simulink model "SF019B_PwrLimr"  (R2013b)
settings: Solver=FixedStepDiscrete  SolverMode=SingleTasking  StartTime=0.0  StopTime=1  FixedStep=0.002  RelTol=1e-3
values from neighbouring files (symbols this model uses):
  ARCHGLBPRM_2MILLISEC_SEC_F32 = DataDict.Constant    [SF019B_PwrLimr_DataDict.m]
  ELECGLBPRM_IVTRCNT_CNT_U08 = DataDict.ConfigParam    [SF019B_PwrLimr_DataDict.m]
  PwrLimrBackEmfConStdT = DataDict.Calibration    [SF019B_PwrLimr_DataDict.m]
  PwrLimrBrdgVltgAdjSlew = DataDict.Calibration    [SF019B_PwrLimr_DataDict.m]
  PwrLimrBrdgVltgAltFltAdj = DataDict.Calibration    [SF019B_PwrLimr_DataDict.m]
  PwrLimrFilAssiRednThd = DataDict.Calibration    [SF019B_PwrLimr_DataDict.m]
  PwrLimrLoVoltAssiRcvrThd = DataDict.Calibration    [SF019B_PwrLimr_DataDict.m]
  PwrLimrLoVoltAssiRcvrTi = DataDict.Calibration    [SF019B_PwrLimr_DataDict.m]
  PWRLIMRMILLISECTOSEC_SECPERMILLISEC_F32 = DataDict.Constant    [SF019B_PwrLimr_DataDict.m]
  PwrLimrMotEnvlpX = DataDict.Calibration    [SF019B_PwrLimr_DataDict.m]
  PwrLimrMotEnvlpY = DataDict.Calibration    [SF019B_PwrLimr_DataDict.m]
  PwrLimrSpdAdjSlewDec = DataDict.Calibration    [SF019B_PwrLimr_DataDict.m]
  PwrLimrSpdAdjSlewEna = DataDict.Calibration    [SF019B_PwrLimr_DataDict.m]
  PwrLimrSpdAdjSlewInc = DataDict.Calibration    [SF019B_PwrLimr_DataDict.m]
  PwrLimrStdOperMotEnvlpX = DataDict.Calibration    [SF019B_PwrLimr_DataDict.m]
  PwrLimrStdOperMotEnvlpY = DataDict.Calibration    [SF019B_PwrLimr_DataDict.m]
  PwrLimrVltgDptMotVelOffsX = DataDict.Calibration    [SF019B_PwrLimr_DataDict.m]
  PwrLimrVltgDptMotVelOffsY = DataDict.Calibration    [SF019B_PwrLimr_DataDict.m]
undefined symbols (not defined in the file or in its folder): D_2MS_SEC_F32
undefined symbols (not defined in the file): ARCHGLBPRM_10MILLISEC_SEC_F32, PwrLimrAssiRednLpFilFrq, PwrLimrMotVelLpFilFrq
libraries: simulink x12, NxtrLim x2
(part 1 of 2)
settings Model: Creator=szj6ld  LastModifiedBy=RZ2YLP
settings SolverCC: AutoInsertRateTranBlk=on  InsertRTBMode=Always
settings DataIOCC: LimitDataPoints=off  SaveFormat=Structure  ReturnWorkspaceOutputs=on
settings OptimizationCC: BlockReduction=off  InlineParams=on  ZeroExternalMemoryAtStartup=off  ZeroInternalMemoryAtStartup=off  OptimizeModelRefInitCode=on  LifeSpan=1
settings DebuggingCC: SignalInfNanChecking=error  SignalRangeChecking=warning  UnderspecifiedInitializationDetection=Simplified  SolverPrmCheckMsg=error  InheritedTsInSrcMsg=error  DiscreteInheritContinuousMsg=error  SingleTaskRateTransMsg=error  TasksWithSamePriorityMsg=error  SigSpecEnsureSampleTimeMsg=error  CheckMatrixSingularityMsg=error  ParameterUnderflowMsg=error  ParameterPrecisionLossMsg=error  ParameterTunabilityLossMsg=error  FixptConstUnderflowMsg=warning  FixptConstOverflowMsg=warning  VectorMatrixConversionMsg=error  SignalLabelMismatchMsg=error  UnconnectedInputMsg=error  UnconnectedOutputMsg=error  UnconnectedLineMsg=error  SFcnCompatibilityMsg=error  UniqueDataStoreMsg=warning  BusObjectLabelMismatch=error  RootOutportRequireBusObject=error  AssertControl=DisableAll  ModelReferenceIOMsg=error  ModelReferenceVersionMismatchMessage=warning  ModelReferenceIOMismatchMessage=error  ModelReferenceCSMismatchMessage=warning  ModelReferenceDataLoggingMessage=error  StateNameClashWarn=warning  StrictBusMsg=ErrorOnBusTreatedAsVector  NonBusSignalsTreatedAsBus=error  SFUnexpectedBacktrackingDiag=error  SFInvalidInputDataAccessInChartInitDiag=error  SFNoUnconditionalDefaultTransitionDiag=error  SFTransitionOutsideNaturalParentDiag=error  SFUnconditionalTransitionShadowingDiag=error  SFUndirectedBroadcastEventsDiag=error
settings ModelReferenceCC: ModelReferenceNumInstancesAllowed=Single
settings RTWCC: SystemTargetFile=autosar.tlc  GenCodeOnly=on  TemplateMakefile=ert_default_tmf  Description=AUTOSAR  GenerateReport=on  ProcessScript=autosar_make_rtw_hook  LaunchReport=on
settings CodeAppCC: GenerateComments=off  IgnoreCustomStorageClasses=off  CustomSymbolStrType=$N$R$M  CustomSymbolStrBlkIO=$N$M  SimulinkBlockComments=off
settings STFCustomTargetCC: ParMdlRefBuildCompliant=on  CompOptLevelCompliant=on  IncludeMdlTerminateFcn=off  CombineOutputUpdateFcns=on  SuppressErrorStatus=on  ERTFirstTimeCompliant=on  ERTCustomFileBanners=on  SupportNonFinite=off  SupportComplex=off  SupportContinuousTime=off  SupportNonInlinedSFcns=off  MATLABClassNameForMDSCustomization=Simulink.SoftwareTarget.ERTCustomization  AutosarCompliant=on  GRTInterface=off  SystemTargetFile=autosar.tlc
settings ERTTargetCC: CodeReplacementLibrary=ANSI_C  ConcurrentExecutionCompliant=off  IncludeMdlTerminateFcn=off  SuppressErrorStatus=on  SupportNonFinite=off  SupportComplex=off  ModelStepFunctionPrototypeControlCompliant=off  CPPClassGenCompliant=off  AutosarCompliant=on  InlinedParameterPlacement=NonHierarchical  ERTCustomFileTemplate=example_file_process.tlc  EnableUserReplacementTypes=on

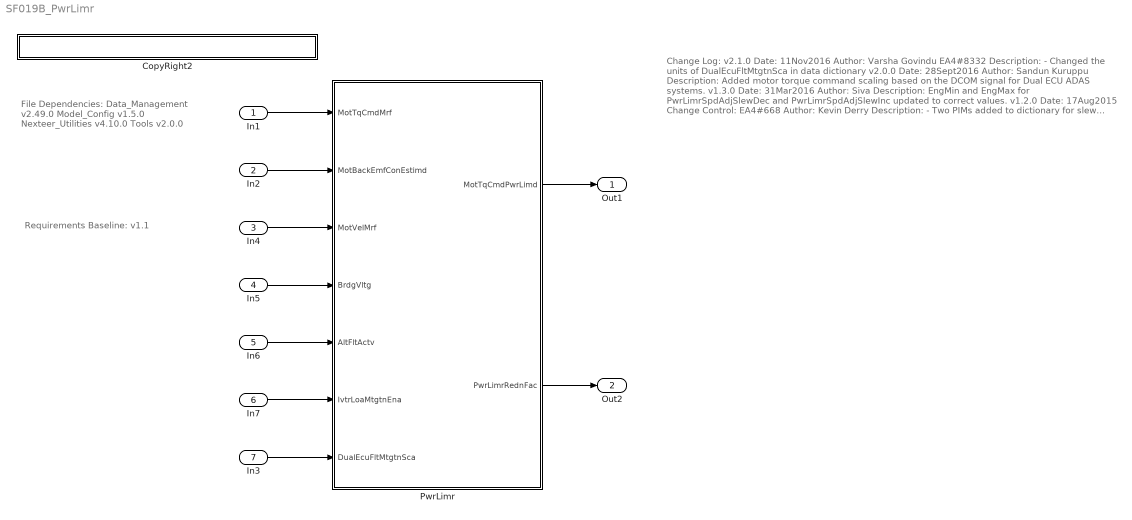
== system SF019B_PwrLimr ==
  note: Requirements Baseline: v1.1
  note: File Dependencies:
      |
      | Data_Management v2.49.0
      | Model_Config v1.5.0
      | Nexteer_Utilities v4.10.0
      | Tools v2.0.0
  note: Change Log:
      |
      | v2.1.0
      | Date: 11Nov2016
      | Author: Varsha Govindu
      | EA4#8332
      | Description:
      | - Changed the units of DualEcuFltMtgtnSca in data dictionary
      |
      | v2.0.0
      | Date: 28Sept2016
      | Author: Sandun Kuruppu
      | Description:
      | Added motor torque command scaling based on the DCOM signal for Dual ECU ADAS systems.
      |
      | v1.3.0
      | Date: 31Mar2016
      | Author: Siva
      | Description:
      | EngMin and EngMax for PwrLimrSpdAdjSlewDec and PwrLimrSpdAdjSlewInc updated to correct values.
      |
      | v1.2.0
      | Date:  17Aug2015
      | Change Control:  EA4#668
      | Author:  Kevin Derry
      | Description:
      | -  Two PIMs added to dictionary for slew operations
      | -  Saturation block added to Per1 output.
      | -  Saturation block added to Per2 output.
      | -  PWRLIMRTQLIMHILIM_CNT_LGC  is now ULS_F32
      | -  PWRLIMRTQLIMLOLIM_CNT_LGC  is now ULS_F32
      | -  Cal PwrLimrVltgDptMotVelOffsY.EngMax was 1350, now 695 to match EA3.
      |
      | v1.1.0
      | Date:  14Aug2015
      | Change Control: EA4#668
      | Author:  Kevin Derry
      | Description:
      | -  Three IRVs added to dictionary
      | -  One PIM added to dictionary for fault timer.
      | -  Timer-related clients added to dictionary.
      | -  Corrected Change Control number in v1.0.0 below.
      |
      |
      | V1.0.0
      | Date: 04AUG2015
      | Change Control: EA4#668
      | Author: Chris Wheatley
      | Description:
      | - Initial Release in EA4
      | - Based on Revision 11.0.0 in EA3
      | - This is a level 0 design model and as such
      |   used only for reference.
  In1 : Inport
  In2 : Inport  Port=2
  In4 : Inport  Port=3
  In5 : Inport  Port=4
  In6 : Inport  Port=5
  In7 : Inport  Port=6
  In3 : Inport  Port=7
  CopyRight2 : Subsystem  Description=|  mask(Copyright Information){none=on}
      | Copyright info block.                                               
      |                                                                     
      | Place copyright information at the top of every subsystem in design.
      mask prompts: none "No parameters"
      mask help: Place copyright information at the top of every subsystem in design.
      mask Display:
      | NxtrConf = 'Nexteer Confidential';
      | 
      | sys = bdroot; %handle for the current model ("system")
      | first = get_param(sys,'Created');
      | first = first(end-3:end);  %year is last four digits
      | 
      | last = get_param(sys,'LastModifiedDate');
      | if isempty(last)
      |     last = datestr(now,'yyyy');
      | else
      |     last = last(end-3:end);
      | end
      | 
      | if strcmp(first,last)
      |     fprintf('%s -- Copyright %s Nexteer',NxtrConf,first)
      | else
      |     fprintf('%s -- %s%s- %s Nexteer',NxtrConf,char(169),first,last)
      | end
  PwrLimr : Subsystem  RequirementInfo="{'linktype_rmi_doors' '0000a532 (/E-STEER Core/SubSystem Specifications/Application Functions/SF019B Power Limit Function- Current Mode)' '#SF019B_245' 'true' 'REQ:  SF019B_245' '' ; 'linktype_rmi_doors' '0000a532 (/E-STEER Core/SubSystem Specifications/Application Functions/SF019B Power Limit Function- Current Mode)' '#SF019B_9' 'true' 'REQ:  SF019B_9' '' ; 'linktype_rmi_doors' '0000a532 (/E-STEER Core/SubSystem Specifications/Application Functions/SF019B Power Limit Function- Current Mode)' '#SF019B_32' 'true' 'REQ:  SF019B_32' '' ; 'linktype_rmi_doors' '0000a532 (/E-STEER Core/SubSystem Specifications/Application Functions/SF019B Power Limit Function- Current Mode)' '#SF019B_33' 'true' 'REQ:  SF019B_33' '' ; 'linktype_rmi_doors' '0000a532 (/E-STEER Core/SubSystem Specifications/Application Functions/SF019B Power Limit Function- Current Mode)' '#SF019B_34' 'true' 'REQ:  SF019B_34' '' ; 'linktype_rmi_doors' '0000a532 (/E-STEER Core/SubSystem Specifications/Application Functions/SF019B Power Limit Function- Current Mode)' '#SF019B_35' 'true' 'REQ:  SF019B_35' '' ; 'linktype_rmi_doors' '0000a532 (/E-STEER Core/SubSystem Specifications/Application Functions/SF019B Power Limit Function- Current Mode)' '#SF019B_36' 'true' 'REQ:  SF019B_36' '' ; 'linktype_rmi_doors' '0000a532 (/E-STEER Core/SubSystem Specifications/Application Functions/SF019B Power Limit Function- Current Mode)' '#SF019B_250' 'true' 'REQ:  SF019B_250' '' ; 'linktype_rmi_doors' '0000a532 (/E-STEER Core/SubSystem Specifications/Application Functions/SF019B Power Limit Function- Current Mode)' '#SF019B_11' 'true' 'REQ:  SF019B_11' '' ; 'linktype_rmi_doors' '0000a532 (/E-STEER Core/SubSystem Specifications/Application Functions/SF019B Power Limit Function- Current Mode)' '#SF019B_37' 'true' 'REQ:  SF019B_37' '' } %GIDa_deb22b8e_5f7e_4de5_8336_875e20a00c31"
  Out1 : Outport
  Out2 : Outport  Port=2
  wires:
  In1/1 -> PwrLimr/1(MotTqCmdMrf)
  In2/1 -> PwrLimr/2(MotBackEmfConEstimd)
  In4/1 -> PwrLimr/3(MotVelMrf)
  In5/1 -> PwrLimr/4(BrdgVltg)
  In6/1 -> PwrLimr/5(AltFltActv)
  In7/1 -> PwrLimr/6(IvtrLoaMtgtnEna)
  PwrLimr/1(MotTqCmdPwrLimd) -> Out1/1
  PwrLimr/2(PwrLimrRednFac) -> Out2/1
  In3/1 -> PwrLimr/7(DualEcuFltMtgtnSca)

== system SF019B_PwrLimr/CopyRight2 ==

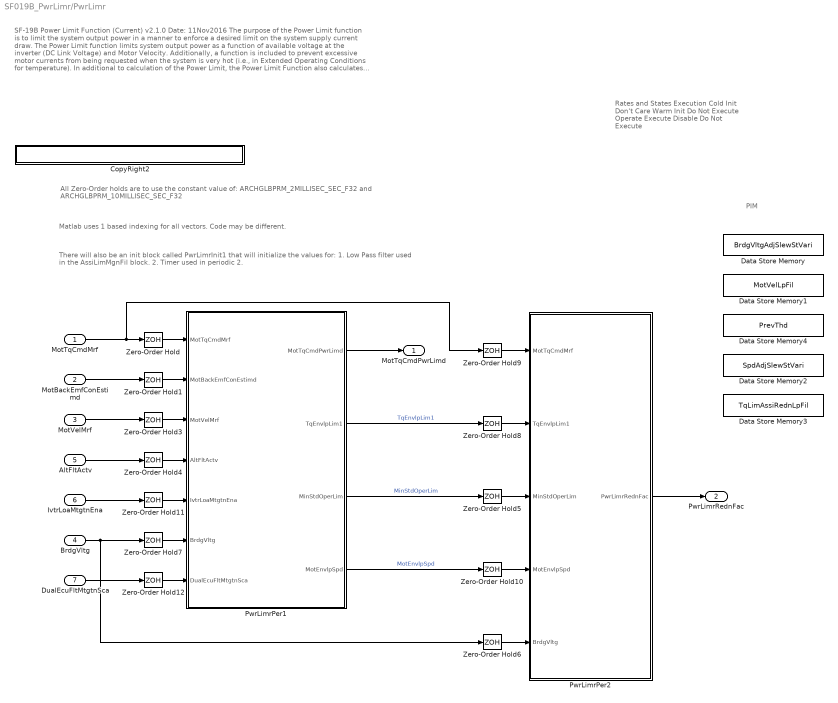
== system SF019B_PwrLimr/PwrLimr ==
  note: Matlab uses 1 based indexing for all vectors. Code may be different.
  note: There will also be an init block called PwrLimrInit1 that will initialize the values for:
      |    1. Low Pass filter used in the AssiLimMgnFil block.
      |    2. Timer used in periodic 2.
  note: SF-19B Power Limit Function (Current)
      | v2.1.0 Date: 11Nov2016
      |
      | The purpose of the Power Limit function is to limit the system output  power in a manner to enforce a desired limit on the system supply current draw.
      | The Power Limit function limits system output power as a function of available voltage at the inverter (DC Link Voltage) and Motor Velocity.  Additionally,
      | a function is included to prevent excessive  motor currents from being requested when the system is very hot (i.e., in Extended Operating Conditions
      | for temperature).
      | In additional to calculation of the Power Limit, the Power Limit Function  also calculates a level of degradation from Standard Operating Conditions full
      | performance and sets flags appropriately for a DTC (Log Only).
  note: Rates and States Execution
      |   Cold Init     Don't Care
      |   Warm Init   Do Not Execute
      |   Operate     Execute
      |   Disable      Do Not Execute
  note: All Zero-Order holds are to use the constant value of:
      | ARCHGLBPRM_2MILLISEC_SEC_F32 and  ARCHGLBPRM_10MILLISEC_SEC_F32
  note: PIM
  MotTqCmdMrf : Inport  RequirementInfo="{}  %GIDa_a11c376a_47bf_4292_9658_09aa228911af"
  MotBackEmfConEstimd : Inport  Port=2
  MotVelMrf : Inport  Port=3
  BrdgVltg : Inport  Port=4
  AltFltActv : Inport  Port=5
  IvtrLoaMtgtnEna : Inport  Port=6
  DualEcuFltMtgtnSca : Inport  Port=7
  CopyRight2 : Subsystem  Description=|  mask(Copyright Information){none=on}
      | Copyright info block.                                               
      |                                                                     
      | Place copyright information at the top of every subsystem in design.
      mask prompts: none "No parameters"
      mask help: Place copyright information at the top of every subsystem in design.
      mask Display:
      | NxtrConf = 'Nexteer Confidential';
      | 
      | sys = bdroot; %handle for the current model ("system")
      | first = get_param(sys,'Created');
      | first = first(end-3:end);  %year is last four digits
      | 
      | last = get_param(sys,'LastModifiedDate');
      | if isempty(last)
      |     last = datestr(now,'yyyy');
      | else
      |     last = last(end-3:end);
      | end
      | 
      | if strcmp(first,last)
      |     fprintf('%s -- Copyright %s Nexteer',NxtrConf,first)
      | else
      |     fprintf('%s -- %s%s- %s Nexteer',NxtrConf,char(169),first,last)
      | end
  Data Store Memory : DataStoreMemory  DataStoreName=BrdgVltgAdjSlewStVari  ReadBeforeWriteMsg=warning  WriteAfterWriteMsg=warning  WriteAfterReadMsg=warning  StateMustResolveToSignalObject=on
  Data Store Memory1 : DataStoreMemory  DataStoreName=MotVelLpFil  ReadBeforeWriteMsg=warning  WriteAfterWriteMsg=warning  WriteAfterReadMsg=warning  InitialValue=[]  OutDataTypeStr=Bus: FilLpRec1  StateMustResolveToSignalObject=on
  Data Store Memory2 : DataStoreMemory  DataStoreName=SpdAdjSlewStVari  ReadBeforeWriteMsg=warning  WriteAfterWriteMsg=warning  WriteAfterReadMsg=warning  StateMustResolveToSignalObject=on
  Data Store Memory3 : DataStoreMemory  DataStoreName=TqLimAssiRednLpFil  ReadBeforeWriteMsg=warning  WriteAfterWriteMsg=warning  WriteAfterReadMsg=warning  InitialValue=[]  OutDataTypeStr=Bus: FilLpRec1  StateMustResolveToSignalObject=on
  Data Store Memory4 : DataStoreMemory  DataStoreName=PrevThd  ReadBeforeWriteMsg=warning  WriteAfterWriteMsg=warning  WriteAfterReadMsg=warning  StateMustResolveToSignalObject=on
  PwrLimrPer1 : Subsystem  RequirementInfo="{'linktype_rmi_doors' '0000a532 (/E-STEER Core/SubSystem Specifications/Application Functions/SF019B Power Limit Function- Current Mode)' '#SF019B_197' 'true' 'REQ:  SF019B_197' '' ; 'linktype_rmi_doors' '0000a532 (/E-STEER Core/SubSystem Specifications/Application Functions/SF019B Power Limit Function- Current Mode)' '#SF019B_198' 'true' 'REQ:  SF019B_198' '' ; 'linktype_rmi_doors' '0000a532 (/E-STEER Core/SubSystem Specifications/Application Functions/SF019B Power Limit Function- Current Mode)' '#SF019B_199' 'true' 'REQ:  SF019B_199' '' ; 'linktype_rmi_doors' '0000a532 (/E-STEER Core/SubSystem Specifications/Application Functions/SF019B Power Limit Function- Current Mode)' '#SF019B_200' 'true' 'REQ:  SF019B_200' '' ; 'linktype_rmi_doors' '0000a532 (/E-STEER Core/SubSystem Specifications/Application Functions/SF019B Power Limit Function- Current Mode)' '#SF019B_254' 'true' 'REQ:  SF019B_254' '' ; 'linktype_rmi_doors' '0000a532 (/E-STEER Core/SubSystem Specifications/Application Functions/SF019B Power Limit Function- Current Mode)' '#SF019B_192' 'true' 'REQ:  SF019B_192' '' } %GIDa_bc7142bf_0b54_4f48_97b6_48859e905753"
  PwrLimrPer2 : Subsystem  RequirementInfo="{'linktype_rmi_doors' '0000a532 (/E-STEER Core/SubSystem Specifications/Application Functions/SF019B Power Limit Function- Current Mode)' '#SF019B_193' 'true' 'REQ:  SF019B_193' '' } %GIDa_9316d20a_733a_4c44_a986_53eaf77b60cd"
  Zero-Order Hold{,1,3..11} (11 alike) : ZeroOrderHold  SampleTime=-1
  Zero-Order Hold12 : ZeroOrderHold  SampleTime=D_2MS_SEC_F32
  MotTqCmdPwrLimd : Outport
  PwrLimrRednFac : Outport  Port=2
  wires:
  PwrLimrPer1/1(MotTqCmdPwrLimd) -> MotTqCmdPwrLimd/1
  PwrLimrPer1/3(MinStdOperLim) -> Zero-Order Hold5/1  "MinStdOperLim"
  MotBackEmfConEstimd/1 -> Zero-Order Hold1/1
  PwrLimrPer2/1(PwrLimrRednFac) -> PwrLimrRednFac/1
  MotVelMrf/1 -> Zero-Order Hold3/1
  BrdgVltg/1 -> Zero-Order Hold7/1, Zero-Order Hold6/1
  Zero-Order Hold1/1 -> PwrLimrPer1/2(MotBackEmfConEstimd)
  Zero-Order Hold3/1 -> PwrLimrPer1/3(MotVelMrf)
  Zero-Order Hold7/1 -> PwrLimrPer1/6(BrdgVltg)
  Zero-Order Hold9/1 -> PwrLimrPer2/1(MotTqCmdMrf)
  Zero-Order Hold8/1 -> PwrLimrPer2/2(TqEnvlpLim1)
  Zero-Order Hold5/1 -> PwrLimrPer2/3(MinStdOperLim)
  Zero-Order Hold6/1 -> PwrLimrPer2/5(BrdgVltg)
  Zero-Order Hold/1 -> PwrLimrPer1/1(MotTqCmdMrf)
  MotTqCmdMrf/1 -> Zero-Order Hold9/1, Zero-Order Hold/1
  Zero-Order Hold10/1 -> PwrLimrPer2/4(MotEnvlpSpd)
  PwrLimrPer1/4(MotEnvlpSpd) -> Zero-Order Hold10/1  "MotEnvlpSpd"
  PwrLimrPer1/2(TqEnvlpLim1) -> Zero-Order Hold8/1  "TqEnvlpLim1"
  AltFltActv/1 -> Zero-Order Hold4/1
  Zero-Order Hold4/1 -> PwrLimrPer1/4(AltFltActv)
  IvtrLoaMtgtnEna/1 -> Zero-Order Hold11/1
  Zero-Order Hold11/1 -> PwrLimrPer1/5(IvtrLoaMtgtnEna)
  Zero-Order Hold12/1 -> PwrLimrPer1/7(DualEcuFltMtgtnSca)
  DualEcuFltMtgtnSca/1 -> Zero-Order Hold12/1

== system SF019B_PwrLimr/PwrLimr/CopyRight2 ==

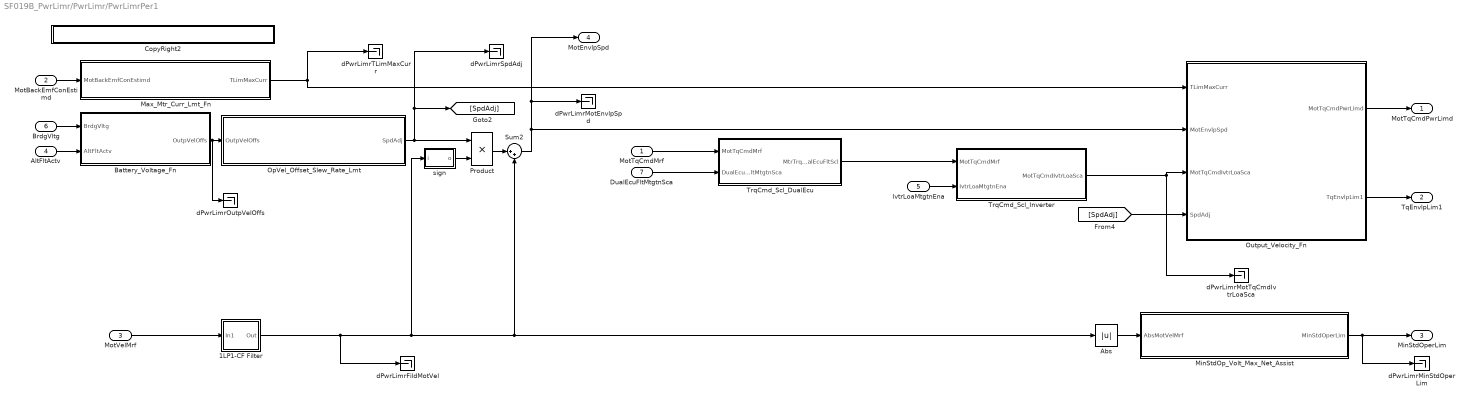
== system SF019B_PwrLimr/PwrLimr/PwrLimrPer1 ==
  MotTqCmdMrf : Inport
  MotBackEmfConEstimd : Inport  Port=2
  MotVelMrf : Inport  Port=3
  AltFltActv : Inport  Port=4
  IvtrLoaMtgtnEna : Inport  Port=5
  BrdgVltg : Inport  Port=6
  DualEcuFltMtgtnSca : Inport  Port=7
  1LP1-CF Filter : Subsystem  RequirementInfo="{'linktype_rmi_doors' '0000a532 (/E-STEER Core/SubSystem Specifications/Application Functions/SF019B Power Limit Function- Current Mode)' '#SF019B_130' 'true' 'REQ:  SF019B_130' '' ; 'linktype_rmi_doors' '0000a532 (/E-STEER Core/SubSystem Specifications/Application Functions/SF019B Power Limit Function- Current Mode)' '#SF019B_131' 'true' 'REQ:  SF019B_131' '' } %GIDa_0c73a69f_0b65_451d_a3dd_7bbd8b392771"  mask(1LP1-CF Filter){Ts=ARCHGLBPRM_2MILLISEC_SEC_F32, Kn_Hz=PwrLimrMotVelLpFilFrq, IC=0}
      mask prompts: Ts "Function Time Step (seconds)"; Kn_Hz "Cutoff Frequency in Hz"; IC "Initial Condition (Enineering Units)"
      mask help: version: Jun 14, 2012
      mask init:
      | %Convert cutoff frequency from Hz into floating point "counts"
      | Kn_Cnt = 1-exp(-2*pi*Kn_Hz*Ts);
      | 
      | %Filter design document originally called this value Knum
      | Knum = Kn_Cnt;
      settings: AttributesFormatString=%<Kn_Hz>
      mask Display:
      | port_label('input',1,'y')
      | disp 'LPF'
      | 
      | %a = [2:0.1:5.2]';
      | %b = sin(2*a);
      | %c = 0.7*sin(25*a);
      | %d = b+c;
      | %e = vertcat(d, b);
      | %plot(e);
  Abs : Abs
  Battery_Voltage_Fn : Subsystem  RequirementInfo="{'linktype_rmi_doors' '0000a532 (/E-STEER Core/SubSystem Specifications/Application Functions/SF019B Power Limit Function- Current Mode)' '#SF019B_64' 'true' 'REQ:  SF019B_64' '' ; 'linktype_rmi_doors' '0000a532 (/E-STEER Core/SubSystem Specifications/Application Functions/SF019B Power Limit Function- Current Mode)' '#SF019B_71' 'true' 'REQ:  SF019B_71' '' ; 'linktype_rmi_doors' '0000a532 (/E-STEER Core/SubSystem Specifications/Application Functions/SF019B Power Limit Function- Current Mode)' '#SF019B_202' 'true' 'REQ:  SF019B_202' '' } %GIDa_d1728748_224a_4c27_968a_5f2e6b163336"
  CopyRight2 : Subsystem  Description=|  mask(Copyright Information){none=on}
      | Copyright info block.                                               
      |                                                                     
      | Place copyright information at the top of every subsystem in design.
      mask prompts: none "No parameters"
      mask help: Place copyright information at the top of every subsystem in design.
      mask Display:
      | NxtrConf = 'Nexteer Confidential';
      | 
      | sys = bdroot; %handle for the current model ("system")
      | first = get_param(sys,'Created');
      | first = first(end-3:end);  %year is last four digits
      | 
      | last = get_param(sys,'LastModifiedDate');
      | if isempty(last)
      |     last = datestr(now,'yyyy');
      | else
      |     last = last(end-3:end);
      | end
      | 
      | if strcmp(first,last)
      |     fprintf('%s -- Copyright %s Nexteer',NxtrConf,first)
      | else
      |     fprintf('%s -- %s%s- %s Nexteer',NxtrConf,char(169),first,last)
      | end
  Max_Mtr_Curr_Lmt_Fn : Subsystem  RequirementInfo="{'linktype_rmi_doors' '0000a532 (/E-STEER Core/SubSystem Specifications/Application Functions/SF019B Power Limit Function- Current Mode)' '#SF019B_223' 'true' 'REQ:  SF019B_223' '' ; 'linktype_rmi_doors' '0000a532 (/E-STEER Core/SubSystem Specifications/Application Functions/SF019B Power Limit Function- Current Mode)' '#SF019B_228' 'true' 'REQ:  SF019B_228' '' } %GIDa_6b055ca6_9043_4c99_8b1e_e40a2fd42a97"
  MinStdOp_Volt_Max_Net_Assist : Subsystem  RequirementInfo="{'linktype_rmi_doors' '0000a532 (/E-STEER Core/SubSystem Specifications/Application Functions/SF019B Power Limit Function- Current Mode)' '#SF019B_181' 'true' 'REQ:  SF019B_181' '' } %GIDa_2f9662a2_e8f7_41b7_8f97_97adeb7707be"
  OpVel_Offset_Slew_Rate_Lmt : Subsystem  RequirementInfo="{'linktype_rmi_doors' '0000a532 (/E-STEER Core/SubSystem Specifications/Application Functions/SF019B Power Limit Function- Current Mode)' '#SF019B_109' 'true' 'REQ:  SF019B_109' '' ; 'linktype_rmi_doors' '0000a532 (/E-STEER Core/SubSystem Specifications/Application Functions/SF019B Power Limit Function- Current Mode)' '#SF019B_204' 'true' 'REQ:  SF019B_204' '' ; 'linktype_rmi_doors' '0000a532 (/E-STEER Core/SubSystem Specifications/Application Functions/SF019B Power Limit Function- Current Mode)' '#SF019B_119' 'true' 'REQ:  SF019B_119' '' } %GIDa_909babbb_53a9_45aa_87ad_ec816ad605cc"
  Output_Velocity_Fn : Subsystem  RequirementInfo="{'linktype_rmi_doors' '0000a532 (/E-STEER Core/SubSystem Specifications/Application Functions/SF019B Power Limit Function- Current Mode)' '#SF019B_140' 'true' 'REQ:  SF019B_140' '' ; 'linktype_rmi_doors' '0000a532 (/E-STEER Core/SubSystem Specifications/Application Functions/SF019B Power Limit Function- Current Mode)' '#SF019B_141' 'true' 'REQ:  SF019B_141' '' ; 'linktype_rmi_doors' '0000a532 (/E-STEER Core/SubSystem Specifications/Application Functions/SF019B Power Limit Function- Current Mode)' '#SF019B_142' 'true' 'REQ:  SF019B_142' '' ; 'linktype_rmi_doors' '0000a532 (/E-STEER Core/SubSystem Specifications/Application Functions/SF019B Power Limit Function- Current Mode)' '#SF019B_163' 'true' 'REQ:  SF019B_163' '' ; 'linktype_rmi_doors' '0000a532 (/E-STEER Core/SubSystem Specifications/Application Functions/SF019B Power Limit Function- Current Mode)' '#SF019B_164' 'true' 'REQ:  SF019B_164' '' ; 'linktype_rmi_doors' '0000a532 (/E-STEER Core/SubSystem Specifications/Application Functions/SF019B Power Limit Function- Current Mode)' '#SF019B_165' 'true' 'REQ:  SF019B_165' '' ; 'linktype_rmi_doors' '0000a532 (/E-STEER Core/SubSystem Specifications/Application Functions/SF019B Power Limit Function- Current Mode)' '#SF019B_166' 'true' 'REQ:  SF019B_166' '' ; 'linktype_rmi_doors' '0000a532 (/E-STEER Core/SubSystem Specifications/Application Functions/SF019B Power Limit Function- Current Mode)' '#SF019B_167' 'true' 'REQ:  SF019B_167' '' ; 'linktype_rmi_doors' '0000a532 (/E-STEER Core/SubSystem Specifications/Application Functions/SF019B Power Limit Function- Current Mode)' '#SF019B_168' 'true' 'REQ:  SF019B_168' '' ; 'linktype_rmi_doors' '0000a532 (/E-STEER Core/SubSystem Specifications/Application Functions/SF019B Power Limit Function- Current Mode)' '#SF019B_243' 'true' 'REQ:  SF019B_243' '' } %GIDa_89bd92d3_bb2a_43b0_8e08_08e0b975e2ab"
  Product : Product  RndMeth=Zero
  Sum2 : Sum  RequirementInfo="{'linktype_rmi_doors' '0000a532 (/E-STEER Core/SubSystem Specifications/Application Functions/SF019B Power Limit Function- Current Mode)' '#SF019B_217' 'true' 'REQ:  SF019B_217' '' } %GIDa_3cc951fb_a402_4d78_96d4_4f365f16fbec"  Inputs=|++
  TrqCmd_Scl_DualEcu : Subsystem  RequirementInfo={'linktype_rmi_doors' '0000a532 (/E-STEER Core/SubSystem Specifications/Application Functions/SF019B Power Limit Function- Current Mode)' '#SF019B_253' 'true' 'REQ:SF019B_253' '' } %GIDa_9ec26d6a_a46d_445e_b529_83aca02e6735
  TrqCmd_Scl_Inverter : Subsystem  RequirementInfo="{'linktype_rmi_doors' '0000a532 (/E-STEER Core/SubSystem Specifications/Application Functions/SF019B Power Limit Function- Current Mode)' '#SF019B_205' 'true' 'REQ:  SF019B_205' '' ; 'linktype_rmi_doors' '0000a532 (/E-STEER Core/SubSystem Specifications/Application Functions/SF019B Power Limit Function- Current Mode)' '#SF019B_136' 'true' 'REQ:  SF019B_136' '' ; 'linktype_rmi_doors' '0000a532 (/E-STEER Core/SubSystem Specifications/Application Functions/SF019B Power Limit Function- Current Mode)' '#SF019B_246' 'true' 'REQ:  SF019B_246' '' } %GIDa_29455dfd_33a0_4b2a_ad67_e1b24522a062"
  dPwrLimrFildMotVel : Terminator
  dPwrLimrMinStdOperLim : Terminator
  dPwrLimrMotEnvlpSpd : Terminator
  dPwrLimrMotTqCmdIvtrLoaSca : Terminator
  dPwrLimrOutpVelOffs : Terminator
  dPwrLimrSpdAdj : Terminator
  dPwrLimrTLimMaxCurr : Terminator
  sign : Subsystem  mask(2-state sign){}
      mask help: version: Nov 30, 2012
      mask Help:
      | Input < 0, Output = -1
      | Input = 0, Output = +1
      | Input > 0, Output = +1
      mask Display: disp 'sign'
  MotTqCmdPwrLimd : Outport
  TqEnvlpLim1 : Outport  Port=2
  MinStdOperLim : Outport  Port=3
  MotEnvlpSpd : Outport  Port=4
  wires:
  Output_Velocity_Fn/1(MotTqCmdPwrLimd) -> MotTqCmdPwrLimd/1
  Sum2/1 -> dPwrLimrMotEnvlpSpd/1, MotEnvlpSpd/1, Output_Velocity_Fn/2(MotEnvlpSpd)
  BrdgVltg/1 -> Battery_Voltage_Fn/1(BrdgVltg)
  MotVelMrf/1 -> 1LP1-CF Filter/1(In1)
  MotBackEmfConEstimd/1 -> Max_Mtr_Curr_Lmt_Fn/1(MotBackEmfConEstimd)
  Battery_Voltage_Fn/1(OutpVelOffs) -> dPwrLimrOutpVelOffs/1, OpVel_Offset_Slew_Rate_Lmt/1(OutpVelOffs)
  MinStdOp_Volt_Max_Net_Assist/1(MinStdOperLim) -> MinStdOperLim/1, dPwrLimrMinStdOperLim/1
  OpVel_Offset_Slew_Rate_Lmt/1(SpdAdj) -> Product/1, [SpdAdj], dPwrLimrSpdAdj/1
  Abs/1 -> MinStdOp_Volt_Max_Net_Assist/1(AbsMotVelMrf)
  Max_Mtr_Curr_Lmt_Fn/1(TLimMaxCurr) -> dPwrLimrTLimMaxCurr/1, Output_Velocity_Fn/1(TLimMaxCurr)
  Output_Velocity_Fn/2(TqEnvlpLim1) -> TqEnvlpLim1/1
  sign/1(o) -> Product/2
  Product/1 -> Sum2/1
  1LP1-CF Filter/1(Out) -> dPwrLimrFildMotVel/1, sign/1(i), Sum2/2, Abs/1
  AltFltActv/1 -> Battery_Voltage_Fn/2(AltFltActv)
  [SpdAdj] -> Output_Velocity_Fn/4(SpdAdj)
  TrqCmd_Scl_Inverter/1(MotTqCmdIvtrLoaSca) -> Output_Velocity_Fn/3(MotTqCmdIvtrLoaSca), dPwrLimrMotTqCmdIvtrLoaSca/1
  IvtrLoaMtgtnEna/1 -> TrqCmd_Scl_Inverter/2(IvtrLoaMtgtnEna)
  TrqCmd_Scl_DualEcu/1(MtrTrqCmdDualEcuFltScl) -> TrqCmd_Scl_Inverter/1(MotTqCmdMrf)
  MotTqCmdMrf/1 -> TrqCmd_Scl_DualEcu/1(MotTqCmdMrf)
  DualEcuFltMtgtnSca/1 -> TrqCmd_Scl_DualEcu/2(DualEcuFltMtgtnSca)

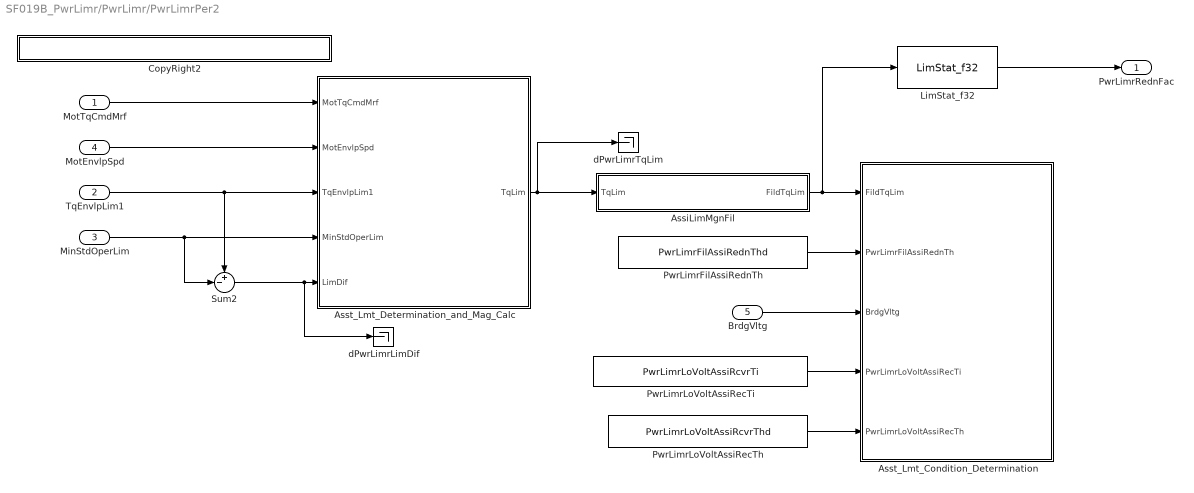
== system SF019B_PwrLimr/PwrLimr/PwrLimrPer2 ==
  MotTqCmdMrf : Inport
  TqEnvlpLim1 : Inport  Port=2
  MinStdOperLim : Inport  Port=3
  MotEnvlpSpd : Inport  Port=4
  BrdgVltg : Inport  Port=5
  AssiLimMgnFil : Subsystem  RequirementInfo="{'linktype_rmi_doors' '0000a532 (/E-STEER Core/SubSystem Specifications/Application Functions/SF019B Power Limit Function- Current Mode)' '#SF019B_89' 'true' 'REQ:  SF019B_89' '' ; 'linktype_rmi_doors' '0000a532 (/E-STEER Core/SubSystem Specifications/Application Functions/SF019B Power Limit Function- Current Mode)' '#SF019B_90' 'true' 'REQ:  SF019B_90' '' } %GIDa_7e36da5d_3e1e_483d_822c_00a07e3a15e0"
  Asst_Lmt_Condition_Determination : Subsystem  RequirementInfo="{'linktype_rmi_doors' '0000a532 (/E-STEER Core/SubSystem Specifications/Application Functions/SF019B Power Limit Function- Current Mode)' '#SF019B_96' 'true' 'REQ:  SF019B_96' '' ; 'linktype_rmi_doors' '0000a532 (/E-STEER Core/SubSystem Specifications/Application Functions/SF019B Power Limit Function- Current Mode)' '#SF019B_97' 'true' 'REQ:  SF019B_97' '' ; 'linktype_rmi_doors' '0000a532 (/E-STEER Core/SubSystem Specifications/Application Functions/SF019B Power Limit Function- Current Mode)' '#SF019B_98' 'true' 'REQ:  SF019B_98' '' ; 'linktype_rmi_doors' '0000a532 (/E-STEER Core/SubSystem Specifications/Application Functions/SF019B Power Limit Function- Current Mode)' '#SF019B_99' 'true' 'REQ:  SF019B_99' '' ; 'linktype_rmi_doors' '0000a532 (/E-STEER Core/SubSystem Specifications/Application Functions/SF019B Power Limit Function- Current Mode)' '#SF019B_100' 'true' 'REQ:  SF019B_100' '' ; 'linktype_rmi_doors' '0000a532 (/E-STEER Core/SubSystem Specifications/Application Functions/SF019B Power Limit Function- Current Mode)' '#SF019B_254' 'true' 'REQ:  SF019B_254' '' ; 'linktype_rmi_doors' '0000a532 (/E-STEER Core/SubSystem Specifications/Application Functions/SF019B Power Limit Function- Current Mode)' '#SF019B_255' 'true' 'REQ:  SF019B_255' '' ; 'linktype_rmi_doors' '0000a532 (/E-STEER Core/SubSystem Specifications/Application Functions/SF019B Power Limit Function- Current Mode)' '#SF019B_218' 'true' 'REQ:  SF019B_218' '' } %GIDa_60f99230_9745_4da5_bdb2_5cd4f8f19d36"
  Asst_Lmt_Determination_and_Mag_Calc : Subsystem  RequirementInfo="{'linktype_rmi_doors' '0000a532 (/E-STEER Core/SubSystem Specifications/Application Functions/SF019B Power Limit Function- Current Mode)' '#SF019B_201' 'true' 'REQ:  SF019B_201' '' } %GIDa_7c94948f_5639_4210_96cd_477abc41e068"
  CopyRight2 : Subsystem  Description=|  mask(Copyright Information){none=on}
      | Copyright info block.                                               
      |                                                                     
      | Place copyright information at the top of every subsystem in design.
      mask prompts: none "No parameters"
      mask help: Place copyright information at the top of every subsystem in design.
      mask Display:
      | NxtrConf = 'Nexteer Confidential';
      | 
      | sys = bdroot; %handle for the current model ("system")
      | first = get_param(sys,'Created');
      | first = first(end-3:end);  %year is last four digits
      | 
      | last = get_param(sys,'LastModifiedDate');
      | if isempty(last)
      |     last = datestr(now,'yyyy');
      | else
      |     last = last(end-3:end);
      | end
      | 
      | if strcmp(first,last)
      |     fprintf('%s -- Copyright %s Nexteer',NxtrConf,first)
      | else
      |     fprintf('%s -- %s%s- %s Nexteer',NxtrConf,char(169),first,last)
      | end
  LimStat_f32 : NxtrLim/LimStat_f32  LoLim=PWRLIMRTQLIMLOLIM_ULS_F32  HiLim=PWRLIMRTQLIMHILIM_ULS_F32
      settings: AttributesFormatString=|
      | Low Limit: %<LoLim>
      | High Limit:%<HiLim>
  PwrLimrFilAssiRednTh : Constant  Value=PwrLimrFilAssiRednThd
  PwrLimrLoVoltAssiRecTh : Constant  Value=PwrLimrLoVoltAssiRcvrThd
  PwrLimrLoVoltAssiRecTi : Constant  Value=PwrLimrLoVoltAssiRcvrTi
  Sum2 : Sum  Inputs=+-|
      settings: AttributesFormatString="[The two inputs to the subtract\\nfunction are signed  TrqEnvLmt1\\nand unsigned Min Std Op Limit.\\nThe result of the subtract\\nLimit_Difference) is a signed\\nvalue.]"
  dPwrLimrLimDif : Terminator
  dPwrLimrTqLim : Terminator
  PwrLimrRednFac : Outport
  wires:
  TqEnvlpLim1/1 -> Asst_Lmt_Determination_and_Mag_Calc/3(TqEnvlpLim1), Sum2/1
  Sum2/1 -> Asst_Lmt_Determination_and_Mag_Calc/5(LimDif), dPwrLimrLimDif/1
  MotTqCmdMrf/1 -> Asst_Lmt_Determination_and_Mag_Calc/1(MotTqCmdMrf)
  Asst_Lmt_Determination_and_Mag_Calc/1(TqLim) -> dPwrLimrTqLim/1, AssiLimMgnFil/1(TqLim)
  BrdgVltg/1 -> Asst_Lmt_Condition_Determination/3(BrdgVltg)
  PwrLimrFilAssiRednTh/1 -> Asst_Lmt_Condition_Determination/2(PwrLimrFilAssiRednTh)
  PwrLimrLoVoltAssiRecTh/1 -> Asst_Lmt_Condition_Determination/5(PwrLimrLoVoltAssiRecTh)
  PwrLimrLoVoltAssiRecTi/1 -> Asst_Lmt_Condition_Determination/4(PwrLimrLoVoltAssiRecTi)
  MotEnvlpSpd/1 -> Asst_Lmt_Determination_and_Mag_Calc/2(MotEnvlpSpd)
  MinStdOperLim/1 -> Asst_Lmt_Determination_and_Mag_Calc/4(MinStdOperLim), Sum2/2
  AssiLimMgnFil/1(FildTqLim) -> LimStat_f32/1, Asst_Lmt_Condition_Determination/1(FildTqLim)
  LimStat_f32/1 -> PwrLimrRednFac/1

== system SF019B_PwrLimr/PwrLimr/PwrLimrPer1/1LP1-CF Filter ==
  note: Filter layout from spreadsheet
  note: This Subsystem represents a type 1LP1-CF Low-Pass filter with floating point math. Layout and nomenclature taken from Design Document authored by Mark Colosky.
  note: REVISIONS
      |   Feb 13, 2012.  Date created.
      |   Feb 17, 2012.  Conversion from Hz to Knum moved to Initialization tab of mask dialog box.
      |   Feb 20, 2012.  Parameterized 1/z block Initial Condition instead of hard-coded = 0.
      |   Jun 14, 2012.  Edited Icon to match other 1LP1-CF variants.
  In1 : Inport
  Constant : Constant  Value=Knum
  Integer Delay : Delay  DelayLength=1  InitialCondition=IC  SampleTime=0.002
  Product1 : Product  RndMeth=Zero
  Sum : Sum  Inputs=|+-
  Sum1 : Sum  Inputs=|++
  Out : Outport
  wires:
  Sum1/1 -> Out/1, Integer Delay/1  "e"
  In1/1 -> Sum/1  "Unfiltered_Signal"
  Integer Delay/1 -> Sum/2, Sum1/2  "f"
  Product1/1 -> Sum1/1  "d"
  Constant/1 -> Product1/1
  Sum/1 -> Product1/2  "c"

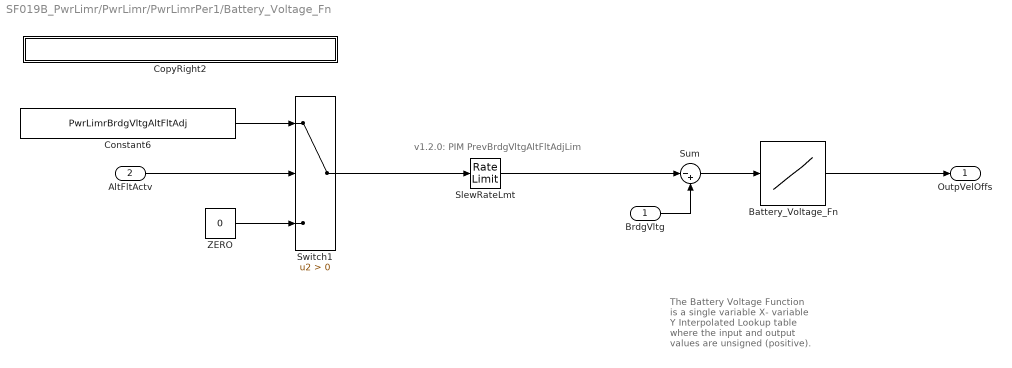
== system SF019B_PwrLimr/PwrLimr/PwrLimrPer1/Battery_Voltage_Fn ==
  note: v1.2.0: PIM PrevBrdgVltgAltFltAdjLim
  note: The Battery Voltage Function is a single variable X-
      | variable Y Interpolated Lookup table where the input
      | and output values are unsigned (positive).
  BrdgVltg : Inport
  AltFltActv : Inport  Port=2
  Battery_Voltage_Fn : Lookup  RequirementInfo="{'linktype_rmi_doors' '0000a532 (/E-STEER Core/SubSystem Specifications/Application Functions/SF019B Power Limit Function- Current Mode)' '#SF019B_72' 'true' 'REQ:  SF019B_72' '' } %GIDa_8b606132_e48c_4ba7_84c4_3f6defec0fc8"  InputValues=PwrLimrVltgDptMotVelOffsX  Table=PwrLimrVltgDptMotVelOffsY  LookUpMeth=Interpolation-Use End Values
      settings: AttributesFormatString=%<InputValues>\n%<Table>
  Constant6 : Constant  Value=PwrLimrBrdgVltgAltFltAdj
  CopyRight2 : Subsystem  Description=|  mask(Copyright Information){none=on}
      | Copyright info block.                                               
      |                                                                     
      | Place copyright information at the top of every subsystem in design.
      mask prompts: none "No parameters"
      mask help: Place copyright information at the top of every subsystem in design.
      mask Display:
      | NxtrConf = 'Nexteer Confidential';
      | 
      | sys = bdroot; %handle for the current model ("system")
      | first = get_param(sys,'Created');
      | first = first(end-3:end);  %year is last four digits
      | 
      | last = get_param(sys,'LastModifiedDate');
      | if isempty(last)
      |     last = datestr(now,'yyyy');
      | else
      |     last = last(end-3:end);
      | end
      | 
      | if strcmp(first,last)
      |     fprintf('%s -- Copyright %s Nexteer',NxtrConf,first)
      | else
      |     fprintf('%s -- %s%s- %s Nexteer',NxtrConf,char(169),first,last)
      | end
  SlewRateLmt : RateLimiter  RequirementInfo="{'linktype_rmi_doors' '0000a532 (/E-STEER Core/SubSystem Specifications/Application Functions/SF019B Power Limit Function- Current Mode)' '#SF019B_67' 'true' 'REQ:  SF019B_67' '' ; 'linktype_rmi_doors' '0000a532 (/E-STEER Core/SubSystem Specifications/Application Functions/SF019B Power Limit Function- Current Mode)' '#SF019B_210' 'true' 'REQ:  SF019B_210' '' } %GIDa_7229e5e5_0333_4d31_8d0d_02453ff6e772"  RisingSlewLimit=PwrLimrBrdgVltgAdjSlew  FallingSlewLimit=-PwrLimrBrdgVltgAdjSlew  SampleTimeMode=inherited
      settings: AttributesFormatString=+/- %<RisingSlewLimit>
  Sum : Sum  RequirementInfo="{'linktype_rmi_doors' '0000a532 (/E-STEER Core/SubSystem Specifications/Application Functions/SF019B Power Limit Function- Current Mode)' '#SF019B_72' 'true' 'REQ:  SF019B_72' '' } %GIDa_6871de2c_5a63_4d77_88b0_2bf7afa0af25"  Inputs=|-+
  Switch1 : Switch  RequirementInfo="{'linktype_rmi_doors' '0000a532 (/E-STEER Core/SubSystem Specifications/Application Functions/SF019B Power Limit Function- Current Mode)' '#SF019B_71' 'true' 'REQ:  SF019B_71' '' ; 'linktype_rmi_doors' '0000a532 (/E-STEER Core/SubSystem Specifications/Application Functions/SF019B Power Limit Function- Current Mode)' '#SF019B_202' 'true' 'REQ:  SF019B_202' '' } %GIDa_3a71ea55_97bb_4e48_a170_13bdb3bdb514"  Criteria=u2 > Threshold
  ZERO : Constant  Value=0
  OutpVelOffs : Outport
  wires:
  Battery_Voltage_Fn/1 -> OutpVelOffs/1
  AltFltActv/1 -> Switch1/2
  Switch1/1 -> SlewRateLmt/1
  Sum/1 -> Battery_Voltage_Fn/1
  BrdgVltg/1 -> Sum/2
  Constant6/1 -> Switch1/1
  ZERO/1 -> Switch1/3
  SlewRateLmt/1 -> Sum/1

== system SF019B_PwrLimr/PwrLimr/PwrLimrPer1/CopyRight2 ==

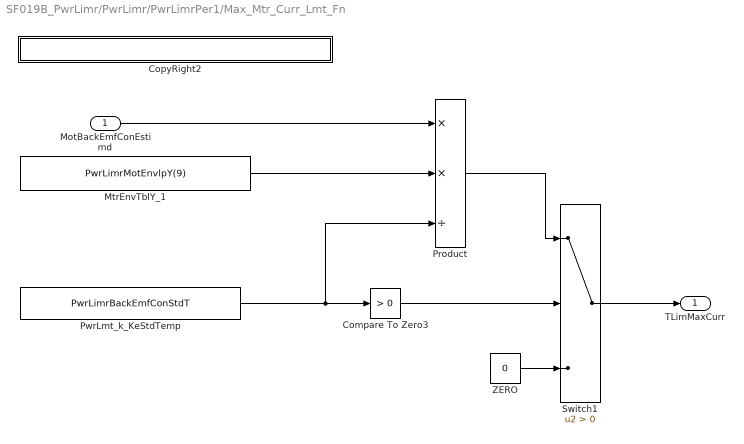
== system SF019B_PwrLimr/PwrLimr/PwrLimrPer1/Max_Mtr_Curr_Lmt_Fn ==
  MotBackEmfConEstimd : Inport
  Compare To Zero3 : simulink/Logic and Bit Operations/Compare To Zero  relop=>  OutDataTypeStr=uint8
  CopyRight2 : Subsystem  Description=|  mask(Copyright Information){none=on}
      | Copyright info block.                                               
      |                                                                     
      | Place copyright information at the top of every subsystem in design.
      mask prompts: none "No parameters"
      mask help: Place copyright information at the top of every subsystem in design.
      mask Display:
      | NxtrConf = 'Nexteer Confidential';
      | 
      | sys = bdroot; %handle for the current model ("system")
      | first = get_param(sys,'Created');
      | first = first(end-3:end);  %year is last four digits
      | 
      | last = get_param(sys,'LastModifiedDate');
      | if isempty(last)
      |     last = datestr(now,'yyyy');
      | else
      |     last = last(end-3:end);
      | end
      | 
      | if strcmp(first,last)
      |     fprintf('%s -- Copyright %s Nexteer',NxtrConf,first)
      | else
      |     fprintf('%s -- %s%s- %s Nexteer',NxtrConf,char(169),first,last)
      | end
  MtrEnvTblY_1 : Constant  Value=PwrLimrMotEnvlpY(9)
      settings: AttributesFormatString="Note :  The (9) denotes the ninth value in the usigned\\nactive Y axis table from the Output Velocity Function."
  Product : Product  Inputs=**/  RndMeth=Zero
  PwrLmt_k_KeStdTemp : Constant  Value=PwrLimrBackEmfConStdT
  Switch1 : Switch  Criteria=u2 > Threshold
      settings: AttributesFormatString=The calculated torque limit from\nthe Maximum Motor Current Limit\nFunction is an unsigned value
  ZERO : Constant  Value=0
  TLimMaxCurr : Outport
  wires:
  PwrLmt_k_KeStdTemp/1 -> Product/3, Compare To Zero3/1
  MtrEnvTblY_1/1 -> Product/2
  MotBackEmfConEstimd/1 -> Product/1
  Compare To Zero3/1 -> Switch1/2
  Product/1 -> Switch1/1
  Switch1/1 -> TLimMaxCurr/1
  ZERO/1 -> Switch1/3

== system SF019B_PwrLimr/PwrLimr/PwrLimrPer1/MinStdOp_Volt_Max_Net_Assist ==
  note: The Minimum Standard Operating Conditions Voltage Maximum Net Assist
      | Function is a single variable X, variable Y Interpolated Lookup table where
      | the input and output values are unsigned (positive).
  AbsMotVelMrf : Inport
  CopyRight2 : Subsystem  Description=|  mask(Copyright Information){none=on}
      | Copyright info block.                                               
      |                                                                     
      | Place copyright information at the top of every subsystem in design.
      mask prompts: none "No parameters"
      mask help: Place copyright information at the top of every subsystem in design.
      mask Display:
      | NxtrConf = 'Nexteer Confidential';
      | 
      | sys = bdroot; %handle for the current model ("system")
      | first = get_param(sys,'Created');
      | first = first(end-3:end);  %year is last four digits
      | 
      | last = get_param(sys,'LastModifiedDate');
      | if isempty(last)
      |     last = datestr(now,'yyyy');
      | else
      |     last = last(end-3:end);
      | end
      | 
      | if strcmp(first,last)
      |     fprintf('%s -- Copyright %s Nexteer',NxtrConf,first)
      | else
      |     fprintf('%s -- %s%s- %s Nexteer',NxtrConf,char(169),first,last)
      | end
  MinStdOp_Volt_Max_NetAssist : Lookup  InputValues=PwrLimrStdOperMotEnvlpX  Table=PwrLimrStdOperMotEnvlpY  LookUpMeth=Interpolation-Use End Values
      settings: AttributesFormatString=%<InputValues>\n%<Table>
  MinStdOperLim : Outport
  wires:
  AbsMotVelMrf/1 -> MinStdOp_Volt_Max_NetAssist/1
  MinStdOp_Volt_Max_NetAssist/1 -> MinStdOperLim/1

== system SF019B_PwrLimr/PwrLimr/PwrLimrPer1/OpVel_Offset_Slew_Rate_Lmt ==
  note: v1.2.0: PIM PrevSpdAdj
  note: The Offset Output Velocity Slew Rate Limit provides a method to limit
      |  the rate at which the Offset Output Velocity value can change.
      | This is accomplished with a dual rate slew limit function.
      |
      | The slew rate limits can be represented in units of Motor Velocity in rad/sec per Second,
      | or in units of Motor Velocity in units of Rad/Sec per 2 millisecond loop.
      |
      | One additional calibration is included to defeat (bypass) the Offset Output
      | Velocity Slew Rate Limit function.
  OutpVelOffs : Inport
  CopyRight2 : Subsystem  Description=|  mask(Copyright Information){none=on}
      | Copyright info block.                                               
      |                                                                     
      | Place copyright information at the top of every subsystem in design.
      mask prompts: none "No parameters"
      mask help: Place copyright information at the top of every subsystem in design.
      mask Display:
      | NxtrConf = 'Nexteer Confidential';
      | 
      | sys = bdroot; %handle for the current model ("system")
      | first = get_param(sys,'Created');
      | first = first(end-3:end);  %year is last four digits
      | 
      | last = get_param(sys,'LastModifiedDate');
      | if isempty(last)
      |     last = datestr(now,'yyyy');
      | else
      |     last = last(end-3:end);
      | end
      | 
      | if strcmp(first,last)
      |     fprintf('%s -- Copyright %s Nexteer',NxtrConf,first)
      | else
      |     fprintf('%s -- %s%s- %s Nexteer',NxtrConf,char(169),first,last)
      | end
  PwrLmt_SlewEnable : Constant  Value=PwrLimrSpdAdjSlewEna
  SlewRateLmt : RateLimiter  RequirementInfo="{'linktype_rmi_doors' '0000a532 (/E-STEER Core/SubSystem Specifications/Application Functions/SF019B Power Limit Function- Current Mode)' '#SF019B_117' 'true' 'REQ:  SF019B_117' '' } %GIDa_cd9f4766_445d_43cb_a15e_d095819d6102"  RisingSlewLimit=PwrLimrSpdAdjSlewInc  FallingSlewLimit=-PwrLimrSpdAdjSlewDec  SampleTimeMode=inherited
      settings: AttributesFormatString=+ %<RisingSlewLimit>\n %<FallingSlewLimit>
  Switch : Switch  RequirementInfo="{'linktype_rmi_doors' '0000a532 (/E-STEER Core/SubSystem Specifications/Application Functions/SF019B Power Limit Function- Current Mode)' '#SF019B_203' 'true' 'REQ:  SF019B_203' '' ; 'linktype_rmi_doors' '0000a532 (/E-STEER Core/SubSystem Specifications/Application Functions/SF019B Power Limit Function- Current Mode)' '#SF019B_122' 'true' 'REQ:  SF019B_122' '' } %GIDa_5b9ca9d3_edad_404d_b5a0_27007a4b5f48"  Threshold=1
  SpdAdj : Outport
  wires:
  SlewRateLmt/1 -> Switch/1
  Switch/1 -> SpdAdj/1
  OutpVelOffs/1 -> SlewRateLmt/1, Switch/3
  PwrLmt_SlewEnable/1 -> Switch/2

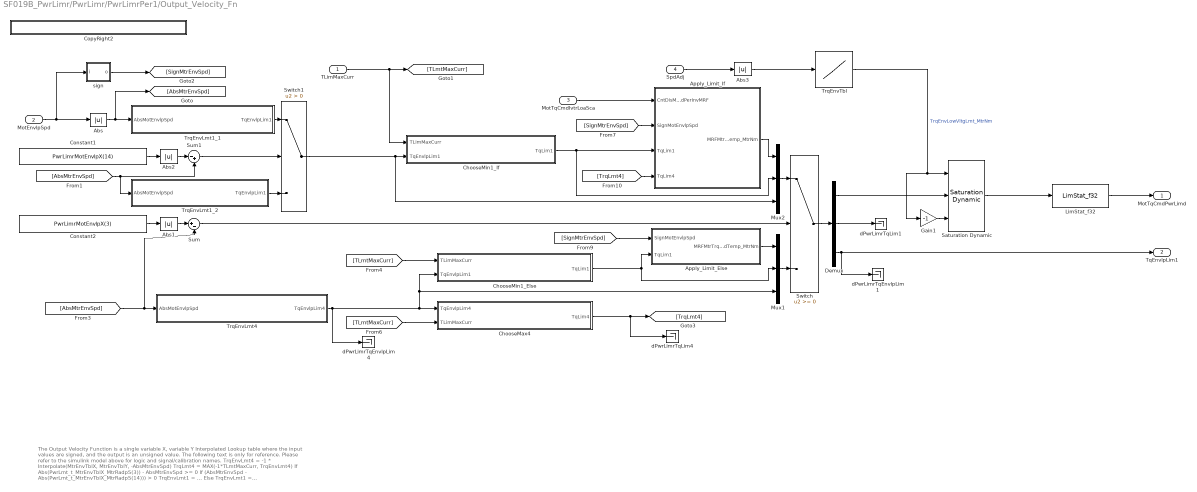
== system SF019B_PwrLimr/PwrLimr/PwrLimrPer1/Output_Velocity_Fn ==
  note: The Output Velocity Function is a single variable X, variable Y Interpolated Lookup table where the input values are signed,
      | and the output is an unsigned value.
      |
      | The following text is only for reference. Please refer to the simulink model above for logic and signal/calibration names.
      |
      | TrqEnvLmt4 = -1 * Interpolate(MtrEnvTblX, MtrEnvTblY, -AbsMtrEnvSpd)
      | TrqLmt4 = MAX(-1*TLmtMaxCurr, TrqEnvLmt4)
      | If Abs(PwrLmt_t_MtrEnvTblX_MtrRadpS(3)) - AbsMtrEnvSpd >= 0
      |     If (AbsMtrEnvSpd - Abs(PwrLmt_t_MtrEnvTblX_MtrRadpS(14))) > 0
      |         TrqEnvLmt1 = ...
      |     Else
      |         TrqEnvLmt1 = Interpolate(MtrEnvTblX, MtrEnvTblY, AbsMtrEnvSpd)
      |     End
      |     TrqLmt1 = MIN(TLmtMaxCurr, TrqEnvLmt1)
      |     MRFMtrTrqCmdTemp = ...
      | Else
      |     TrqEnvLmt1 = TrqEnvLmt4
      |     TrqLmt1 = MIN(TLmtMaxCurr, TrqEnvLmt1)
      |     MRFMtrTrqCmdTemp = ...
      | End
      |
      | TrqEnvLowVltgLmt = Interpolate(MtrEnvTblX, MtrEnvTblY, Abs(SpdAdj))
      | MRFMtrTrqCmd = Limit(MRFMtrTrqCmdTemp, - TrqEnvLowVltgLmt,TrqEnvLowVltgLmt)
  TLimMaxCurr : Inport
  MotEnvlpSpd : Inport  Port=2
  MotTqCmdIvtrLoaSca : Inport  Port=3
  SpdAdj : Inport  Port=4
  Abs{,1..3} (4 alike) : Abs
  Apply_Limit_Else : Subsystem
  Apply_Limit_If : Subsystem
  ChooseMax4 : Subsystem
  ChooseMin1_Else : Subsystem
  ChooseMin1_If : Subsystem
  Constant1 : Constant  Value=PwrLimrMotEnvlpX(14)
  Constant2 : Constant  Value=PwrLimrMotEnvlpX(3)
  CopyRight2 : Subsystem  Description=|  mask(Copyright Information){none=on}
      | Copyright info block.                                               
      |                                                                     
      | Place copyright information at the top of every subsystem in design.
      mask prompts: none "No parameters"
      mask help: Place copyright information at the top of every subsystem in design.
      mask Display:
      | NxtrConf = 'Nexteer Confidential';
      | 
      | sys = bdroot; %handle for the current model ("system")
      | first = get_param(sys,'Created');
      | first = first(end-3:end);  %year is last four digits
      | 
      | last = get_param(sys,'LastModifiedDate');
      | if isempty(last)
      |     last = datestr(now,'yyyy');
      | else
      |     last = last(end-3:end);
      | end
      | 
      | if strcmp(first,last)
      |     fprintf('%s -- Copyright %s Nexteer',NxtrConf,first)
      | else
      |     fprintf('%s -- %s%s- %s Nexteer',NxtrConf,char(169),first,last)
      | end
  Demux : Demux  Outputs=3
  Gain1 : Gain  Gain=-1
  LimStat_f32 : NxtrLim/LimStat_f32  LoLim=SYSGLBPRM_MOTTQCMDLOLIM_MOTNWTMTR_F32  HiLim=SYSGLBPRM_MOTTQCMDHILIM_MOTNWTMTR_F32
      settings: AttributesFormatString=|
      | Low Limit: %<LoLim>
      | High Limit:%<HiLim>
  Mux1 : Mux  Inputs=3
  Mux2 : Mux  Inputs=3
  Saturation Dynamic : simulink/Discontinuities/Saturation Dynamic  OutMin=[]  OutMax=[]  OutDataTypeStr=Inherit: Same as second input  OutDataType=fixdt(1, 16)  OutScaling=2^-10  DoSatur=off
  Sum : Sum  Inputs=|+-
  Sum1 : Sum  Inputs=|-+
  Switch : Switch
  Switch1 : Switch  Criteria=u2 > Threshold
  TrqEnvLmt1_1 : Subsystem
  TrqEnvLmt1_2 : Subsystem
  TrqEnvLmt4 : Subsystem
  TrqEnvTbl : Lookup  InputValues=PwrLimrStdOperMotEnvlpX  Table=PwrLimrStdOperMotEnvlpY  LookUpMeth=Interpolation-Use End Values
      settings: AttributesFormatString=%<InputValues>\n%<Table>
  dPwrLimrTqEnvlpLim1 : Terminator
  dPwrLimrTqEnvlpLim4 : Terminator
  dPwrLimrTqLim1 : Terminator
  dPwrLimrTqLim4 : Terminator
  sign : Subsystem  mask(2-state sign){}
      mask help: version: Nov 30, 2012
      mask Help:
      | Input < 0, Output = -1
      | Input = 0, Output = +1
      | Input > 0, Output = +1
      mask Display: disp 'sign'
  MotTqCmdPwrLimd : Outport
  TqEnvlpLim1 : Outport  Port=2
  wires:
  Switch1/1 -> ChooseMin1_If/2(TqEnvlpLim1), Mux2/3
  [AbsMtrEnvSpd] -> TrqEnvLmt4/1(AbsMotEnvlpSpd), Sum/2
  [AbsMtrEnvSpd] -> Sum1/2, TrqEnvLmt1_2/1(AbsMotEnvlpSpd)
  Abs/1 -> [AbsMtrEnvSpd], TrqEnvLmt1_1/1(AbsMotEnvlpSpd)
  Switch/1 -> Demux/1
  TrqEnvLmt1_2/1(TqEnvlpLim1) -> Switch1/3
  TrqEnvLmt1_1/1(TqEnvlpLim1) -> Switch1/1
  Sum1/1 -> Switch1/2
  Abs2/1 -> Sum1/1
  Constant1/1 -> Abs2/1
  Sum/1 -> Switch/2
  Abs1/1 -> Sum/1
  Constant2/1 -> Abs1/1
  MotEnvlpSpd/1 -> Abs/1, sign/1(i)
  TLimMaxCurr/1 -> ChooseMin1_If/1(TLimMaxCurr), [TLmtMaxCurr]
  ChooseMax4/1(TqLim4) -> [TrqLmt4], dPwrLimrTqLim4/1
  [TLmtMaxCurr] -> ChooseMax4/2(TLimMaxCurr)
  ChooseMin1_Else/1(TqLim1) -> Apply_Limit_Else/2(TqLim1), Mux1/2
  ChooseMin1_If/1(TqLim1) -> Apply_Limit_If/3(TqLim1), Mux2/2
  sign/1(o) -> [SignMtrEnvSpd]
  MotTqCmdIvtrLoaSca/1 -> Apply_Limit_If/1(CntDisMtrTrqCmdPerInvMRF)
  Apply_Limit_If/1(MRFMtrTrqCmdTemp_MtrNm) -> Mux2/1
  [SignMtrEnvSpd] -> Apply_Limit_Else/1(SignMotEnvlpSpd)
  Apply_Limit_Else/1(MRFMtrTrqCmdTemp_MtrNm) -> Mux1/1
  Mux2/1 -> Switch/1
  Mux1/1 -> Switch/3
  [TLmtMaxCurr] -> ChooseMin1_Else/1(TLimMaxCurr)
  TrqEnvLmt4/1(TqEnvlpLim4) -> ChooseMax4/1(TqEnvlpLim4), Mux1/3, ChooseMin1_Else/2(TqEnvlpLim1), dPwrLimrTqEnvlpLim4/1
  [TrqLmt4] -> Apply_Limit_If/4(TqLim4)
  [SignMtrEnvSpd] -> Apply_Limit_If/2(SignMotEnvlpSpd)
  Demux/2 -> dPwrLimrTqLim1/1
  TrqEnvTbl/1 -> Gain1/1, Saturation Dynamic/1  "TrqEnvLowVltgLmt_MtrNm"
  Gain1/1 -> Saturation Dynamic/3
  Demux/1 -> Saturation Dynamic/2
  Saturation Dynamic/1 -> LimStat_f32/1
  SpdAdj/1 -> Abs3/1
  Abs3/1 -> TrqEnvTbl/1
  LimStat_f32/1 -> MotTqCmdPwrLimd/1
  Demux/3 -> TqEnvlpLim1/1, dPwrLimrTqEnvlpLim1/1

== system SF019B_PwrLimr/PwrLimr/PwrLimrPer1/TrqCmd_Scl_DualEcu ==
  MotTqCmdMrf : Inport
  DualEcuFltMtgtnSca : Inport  Port=2
  CopyRight2 : Subsystem  Description=|  mask(Copyright Information){none=on}
      | Copyright info block.                                               
      |                                                                     
      | Place copyright information at the top of every subsystem in design.
      mask prompts: none "No parameters"
      mask help: Place copyright information at the top of every subsystem in design.
      mask Display:
      | NxtrConf = 'Nexteer Confidential';
      | 
      | sys = bdroot; %handle for the current model ("system")
      | first = get_param(sys,'Created');
      | first = first(end-3:end);  %year is last four digits
      | 
      | last = get_param(sys,'LastModifiedDate');
      | if isempty(last)
      |     last = datestr(now,'yyyy');
      | else
      |     last = last(end-3:end);
      | end
      | 
      | if strcmp(first,last)
      |     fprintf('%s -- Copyright %s Nexteer',NxtrConf,first)
      | else
      |     fprintf('%s -- %s%s- %s Nexteer',NxtrConf,char(169),first,last)
      | end
  Product : Product
  MtrTrqCmdDualEcuFltScl : Outport
  wires:
  DualEcuFltMtgtnSca/1 -> Product/2
  MotTqCmdMrf/1 -> Product/1
  Product/1 -> MtrTrqCmdDualEcuFltScl/1
